simulink model "HEV_BTP_basic_Perfect_PID_17_1_2020"  (R2019a)
settings: Solver=VariableStepAuto  StartTime=0  StopTime=600  RelTol=1e-3
undefined symbols (not defined in the file): f_co, f_co2, f_hc, f_nox, f_tbrake_n_bpt, f_tbrake_t_bpt
libraries: nesl_utility x24, sdl_lib x16, fl_lib x13, simulink x6, autolibshared x1
settings Model: Creator=hp  LastModifiedBy=hp
settings SolverCC: ZeroCrossAlgorithm=Adaptive
settings DataIOCC: ExternalInput=[PedalTime,ThrottlePedal,FrontBrakePedal,RearBrakePedal]  LoadExternalInput=on
settings DebuggingCC: IgnoredZcDiagnostic=none

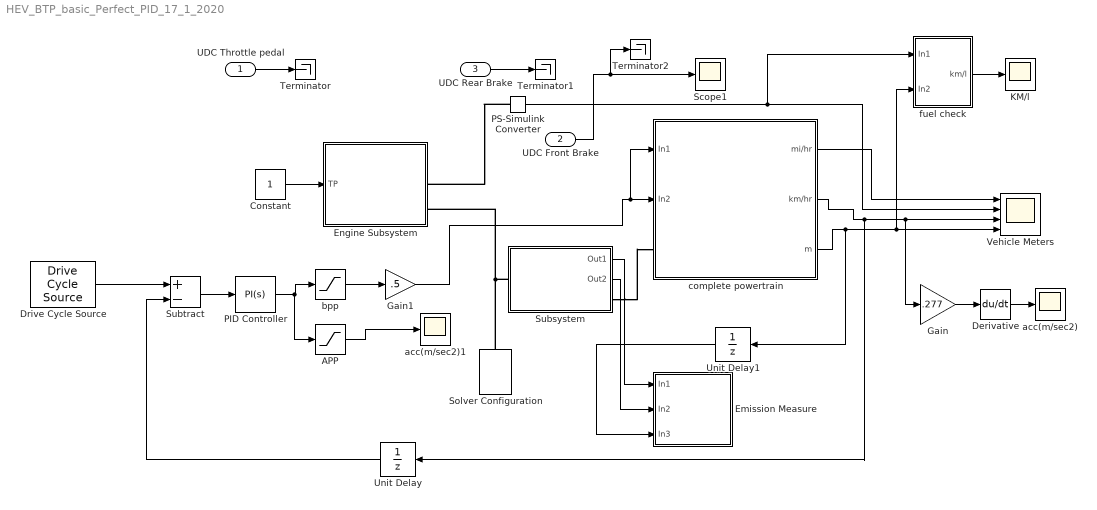
== system HEV_BTP_basic_Perfect_PID_17_1_2020 ==
  UDC Throttle pedal : Inport
  UDC Front Brake : Inport  Port=2
  UDC Rear Brake : Inport  Port=3
  APP : Saturate  UpperLimit=inf  LowerLimit=0
  Constant : Constant
  Derivative : Derivative
  Drive Cycle Source : autolibshared/Drive Cycle Source  cycleVar=US06  fileVar=cycleFTP75.mat  tfinal="600  seconds, Cyclic"  cycleRepeat=on  outAccPort=off  outGearPort=off  gearList=No gear data  t_wot1=5  xdot_woto=0  xdot_wot1=30  t_wot2=20  xdot_wot2=0  t_wotend=30  srcUnit=m/s  outUnit=km/hr  srcAccUnit=m/s/s  outAccUnit=m/s^2  dt=0  aMode=2
      settings: SourceProductName=Powertrain Blockset  SourceProductBaseCode=PW
  Emission Measure : Subsystem
  Engine Subsystem : Subsystem
  Gain : Gain  Gain=.277
  Gain1 : Gain  Gain=.5
  KM/l : Scope
  PID Controller : simulink/Continuous/PID Controller  Controller=PI  Form=Parallel  TimeDomain=Continuous-time  SampleTime=-1  IntegratorMethod=Forward Euler  FilterMethod=Forward Euler  ControllerParametersSource=internal  P=.145  I=.015  D=0  UseFilter=on  N=100  TunerSelectOption=Transfer Function Based (PID Tuner App)  InitialConditionSource=internal  InitialConditionForIntegrator=0  InitialConditionForFilter=0  DifferentiatorICPrevScaledInput=0  ExternalReset=none  TrackingMode=off  Kt=1  LimitOutput=off  UpperSaturationLimit=inf  LowerSaturationLimit=-inf  LinearizeAsGain=on  AntiWindupMode=none  Kb=1  POutMin=[]  POutMax=[]  IOutMin=[]  IOutMax=[]  DOutMin=[]  DOutMax=[]  NOutMin=[]  NOutMax=[]  SumOutMin=[]  SumOutMax=[]  SaturationOutMin=[]  SaturationOutMax=[]  PParamMin=[]  PParamMax=[]  IParamMin=[]  IParamMax=[]  DParamMin=[]  DParamMax=[]  NParamMin=[]  NParamMax=[]  KbParamMin=[]  KbParamMax=[]  KtParamMin=[]  KtParamMax=[]  KbOutMin=[]  KbOutMax=[]  KtOutMin=[]  KtOutMax=[]  IntegratorOutMin=[]  IntegratorOutMax=[]  FilterOutMin=[]  FilterOutMax=[]  SumI1OutMin=[]  SumI1OutMax=[]  SumI2OutMin=[]  SumI2OutMax=[]  SumI3OutMin=[]  SumI3OutMax=[]  SumI4OutMin=[]  SumI4OutMax=[]  SumDOutMin=[]  SumDOutMax=[]  DifferentiatorOutMin=[]  DifferentiatorOutMax=[]  FilterDiffOutCoefMin=[]  FilterDiffOutCoefMax=[]  ReciprocalOutMin=[]  ReciprocalOutMax=[]  SumDenOutMin=[]  SumDenOutMax=[]  SumNumOutMin=[]  SumNumOutMax=[]  DivideOutMin=[]  DivideOutMax=[]  IntegratorContinuousStateAttributes=''  IntegratorStateMustResolveToSignalObject=off  IntegratorRTWStateStorageClass=Auto  FilterContinuousStateAttributes=''  FilterStateMustResolveToSignalObject=off  FilterRTWStateStorageClass=Auto  ParallelPVariant=InternalParameters  IdealPVariant=Disabled  IVariant=InternalParameters  DVariant=Disabled  IntegratorVariant=Continuous  SatVariant=Disabled  AWVariant=Passthrough  PCopyVariant=Disabled  TRVariant=Disabled  FdbkBlocksVariant=Forward  IdealPFdbkVariant=Disabled  SatFdbkVariant=Disabled  DerivativeFilterVariant=Disabled  NVariant=Disabled  NCopyVariant=Disabled_SignalSpec  FilterICVariant=Disabled  IntegratorICVariant=InternalICs  ExternalResetVariant=Disabled  TRSumVariant=Passthrough  SumFdbkVariant=Disabled  SumVariant=Sum_PI
  PS-Simulink Converter : nesl_utility/PS-Simulink Converter  PhysicalDomain=network_engine_domain  SubClassName=ps_output  LeftPortType=input  RightPortType=output  PseudoPeriodic=off  Frequencies=[]  Unit=g/s  AffineConversion=off
  Scope1 : Scope
  Solver Configuration : nesl_utility/Solver Configuration  PhysicalDomain=network_engine_domain  SubClassName=solver  LeftPortType=input  RightPortType=generic  Tones=[]  Harmonics=[]  SimulateNoise=off  Profile=off  UseLocalSampling=off  EnableSwitchedLinearOptims=on  FrequencyDomain=off  UseCCode=off  RelTol=0.001  AbsTol=1e-06  MinStep=1e-09  ToWorkspace=off  RevertToSquareIcSolve=off  NumHomotopyIterations=100  PhasorMode=off  PhasorModeNumHarmonics=1  DoDC=off  ResidualTolerance=1e-09  UseLocalSolver=off  LocalSolverChoice=NE_BACKWARD_EULER_ADVANCER  LocalSolverSampleTime=0.001  DoFixedCost=off  MaxNonlinIter=3  MaxModeIter=2  LinearAlgebra=auto  EquationFormulation=NE_TIME_EF  DelaysMemoryBudget=1024  AutomaticFiltering=on  FilteringTimeConstant=0.001  PartitionStorageMethod=AS_NEEDED  PartitionMemoryBudget=1024  PartitionMethod=ROBUST
  Subsystem : Subsystem
  Subtract : Sum  Inputs=+-
  Terminator : Terminator
  Terminator1 : Terminator
  Terminator2 : Terminator
  Unit Delay : UnitDelay  SampleTime=-1  HasFrameUpgradeWarning=on
  Unit Delay1 : UnitDelay  SampleTime=-1  HasFrameUpgradeWarning=on
  "Vehicle Meters " : Scope  NumInputPorts=4
  acc(m/sec2) : Scope
  acc(m/sec2)1 : Scope
  bpp : Saturate  UpperLimit=0  LowerLimit=-inf
  complete powertrain : Subsystem
  "fuel check " : Subsystem
  wires:
  complete powertrain/2(km/hr) -> Unit Delay/1, "Vehicle Meters "/3, Gain/1
  complete powertrain/1(mi/hr) -> "Vehicle Meters "/1
  complete powertrain/3(m) -> Unit Delay1/1, "Vehicle Meters "/4, "fuel check "/2(In2)
  UDC Front Brake/1 -> Terminator2/1, Scope1/1
  PS-Simulink Converter/1 -> "fuel check "/1(In1), "Vehicle Meters "/2
  Subsystem/2(Out2) -> Emission Measure/2(In2)
  Subsystem/1(Out1) -> Emission Measure/1(In1)
  Unit Delay1/1 -> Emission Measure/3(In3)
  "fuel check "/1(km/l) -> KM/l/1
  Gain/1 -> Derivative/1
  Derivative/1 -> acc(m/sec2)/1
  Drive Cycle Source/1 -> Subtract/1
  Subtract/1 -> PID Controller/1
  PID Controller/1 -> APP/1, bpp/1
  bpp/1 -> Gain1/1
  Gain1/1 -> complete powertrain/1(In1), complete powertrain/2(In2)
  UDC Throttle pedal/1 -> Terminator/1
  UDC Rear Brake/1 -> Terminator1/1
  Unit Delay/1 -> Subtract/2
  APP/1 -> acc(m/sec2)1/1
  Constant/1 -> Engine Subsystem/1(TP)
  connections:
  Solver Configuration/RConn1 -- Engine Subsystem/RConn3 -- Subsystem/LConn1
  PS-Simulink Converter/LConn1 -- Engine Subsystem/RConn2
  Subsystem/RConn1 -- complete powertrain/LConn1

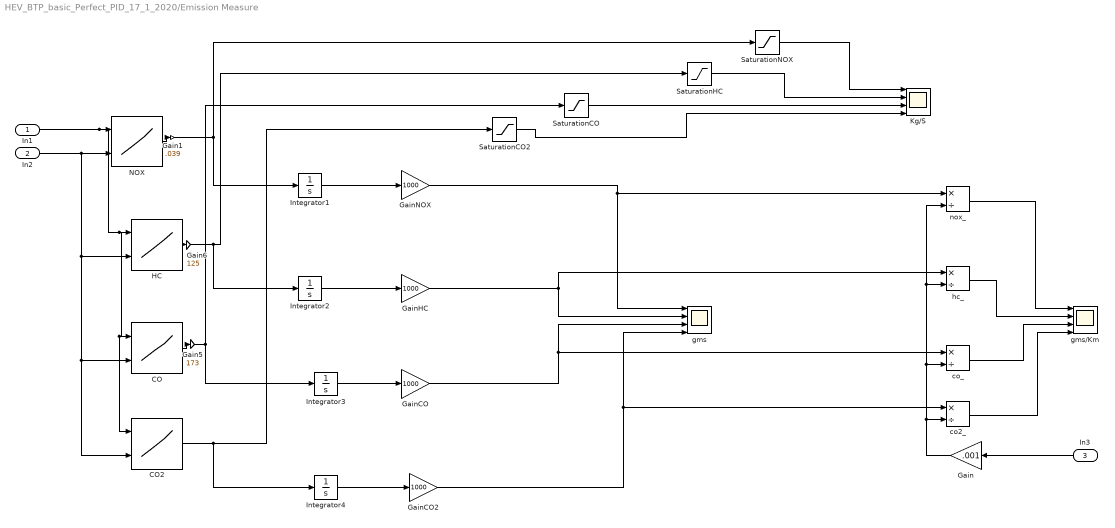
== system HEV_BTP_basic_Perfect_PID_17_1_2020/Emission Measure ==
  In1 : Inport
  In2 : Inport  Port=2
  In3 : Inport  Port=3
  CO : Lookup_n-D  BreakpointsForDimension1=f_tbrake_t_bpt  BreakpointsForDimension2=f_tbrake_n_bpt  Table=f_co  InternalRulePriority=Speed  RndMeth=Simplest  InputSameDT=on
  CO2 : Lookup_n-D  BreakpointsForDimension1=f_tbrake_t_bpt  BreakpointsForDimension2=f_tbrake_n_bpt  Table=f_co2  InternalRulePriority=Speed  RndMeth=Simplest  InputSameDT=on
  Gain : Gain  Gain=.001
  Gain1 : Gain  Gain=.039
  Gain5 : Gain  Gain=173
  Gain6 : Gain  Gain=125
  GainCO : Gain  Gain=1000
  GainCO2 : Gain  Gain=1000
  GainHC : Gain  Gain=1000
  GainNOX : Gain  Gain=1000
  HC : Lookup_n-D  BreakpointsForDimension1=f_tbrake_t_bpt  BreakpointsForDimension2=f_tbrake_n_bpt  Table=f_hc  InternalRulePriority=Speed  RndMeth=Simplest  InputSameDT=on
  Integrator{1..4} (4 alike) : Integrator
  Kg/S : Scope  NumInputPorts=4
  NOX : Lookup_n-D  BreakpointsForDimension1=f_tbrake_t_bpt  BreakpointsForDimension2=f_tbrake_n_bpt  Table=f_nox  InternalRulePriority=Speed  RndMeth=Simplest  InputSameDT=on
  SaturationCO : Saturate  UpperLimit=inf  LowerLimit=0  ZeroCross=off
  SaturationCO2 : Saturate  UpperLimit=inf  LowerLimit=0  ZeroCross=off
  SaturationHC : Saturate  UpperLimit=inf  LowerLimit=0  ZeroCross=off
  SaturationNOX : Saturate  UpperLimit=inf  LowerLimit=0  ZeroCross=off
  co2_ : Product  Inputs=*/
  co_ : Product  Inputs=*/
  gms : Scope  NumInputPorts=4
  gms/Km : Scope  NumInputPorts=4
  hc_ : Product  Inputs=*/
  nox_ : Product  Inputs=*/
  wires:
  NOX/1 -> Gain1/1
  In2/1 -> CO2/2, CO/2, HC/2, NOX/2
  In1/1 -> CO2/1, CO/1, HC/1, NOX/1
  HC/1 -> Gain6/1
  CO/1 -> Gain5/1
  CO2/1 -> SaturationCO2/1, Integrator4/1
  SaturationNOX/1 -> Kg/S/1
  SaturationHC/1 -> Kg/S/2
  SaturationCO2/1 -> Kg/S/4
  SaturationCO/1 -> Kg/S/3
  Gain6/1 -> Integrator2/1, SaturationHC/1
  Gain5/1 -> Integrator3/1, SaturationCO/1
  Integrator3/1 -> GainCO/1
  Integrator4/1 -> GainCO2/1
  Integrator2/1 -> GainHC/1
  Integrator1/1 -> GainNOX/1
  GainCO2/1 -> co2_/1, gms/4
  GainHC/1 -> gms/2, hc_/1
  GainNOX/1 -> nox_/1, gms/1
  GainCO/1 -> gms/3, co_/1
  Gain/1 -> nox_/2, hc_/2, co_/2, co2_/2
  nox_/1 -> gms/Km/1
  hc_/1 -> gms/Km/2
  co_/1 -> gms/Km/3
  co2_/1 -> gms/Km/4
  Gain1/1 -> Integrator1/1, SaturationNOX/1
  In3/1 -> Gain/1

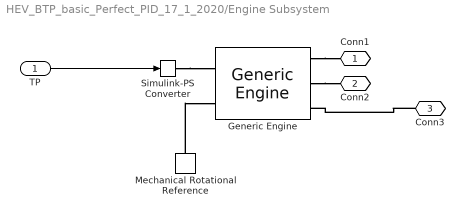
== system HEV_BTP_basic_Perfect_PID_17_1_2020/Engine Subsystem ==
  TP : Inport
  Generic Engine : sdl_lib/Engines/Generic Engine  model_parameterization=1  engine_type=1  P_max=51.5 kW  w_P_max=5500 rpm  w_max=6175 rpm  w_min=500 rpm  w_tab=[500, 1000, 2000, 3000, 4000, 5000, 6000, 7000] rpm  trq_tab=[380, 380, 380, 380, 350, 280, 200, 80] N*m  pwr_tab=[20, 40, 78, 120, 145, 148, 125, 60] kW  interp_method=simscape.enum.interpolation.linear  model_inertia=1  inertia=1 kg*m^2  initial_velocity=875 rpm  model_time_constant=1  time_constant=0.2 s  T0=.01  w_thr=100 rpm  idle_speed=0  idle_speed_reference=875 rpm  tau_controller=1 s  idle_w_thr=1 rpm  redline=0  redline_speed=5000 rpm  tau_redline=1 s  redline_w_thr=1 rpm  fc_model=2  fc_per_rev=22.816 mg/rev  displaced_volume=400 cm^3  rev_per_cycle=2  fc_w_tab=[875, 2000, 3000, 4000, 5000, 6175] rpm  fc_trq_tab=[0, 80, 160, 200, 240, 320, 360, 400] N*m  fc_tab=[0.2, 0.36, 0.56, 0.64, 0.76, 1.08, 1.36, 1.76; 0.4, 0.68, 1.08, 1.24, 1.44, 2, 2.4, 1.96; 0.56, 1.08, 1.6, 1.92, 2.24, 3, 3.4, 4.2; 0.8, 1.44, 2.32, 2.68, 3.2, 4.28, 4.68, 5.32; 1, 1.92, 3.16, 3.76, 4.32, 5.6, 6.48, 7.44; 1.24, 2.4, 4.12, 4.76, 5.52, 7.36, 8.8, 10.6] g/s  bmep_tab=[0, 250, 500, 625, 750, 1000, 1150, 1250] kPa  bsfc_tab=[410, 380, 300, 280, 270, 290, 320, 380; 410, 370, 290, 270, 260, 270, 285, 320; 415, 380, 290, 275, 265, 270, 270, 300; 420, 390, 310, 290, 285, 280, 280, 285; 430, 410, 340, 320, 310, 300, 310, 320; 450, 430, 370, 340, 330, 330, 350, 380] g/hr/kW  fc_interp_method=simscape.enum.interpolation.linear
      settings: SourceProductName=Simscape Driveline  SourceProductBaseCode=LD  LogSimulationData=on
  Mechanical Rotational Reference : fl_lib/Mechanical/Rotational Elements/Mechanical Rotational Reference
  Simulink-PS Converter : nesl_utility/Simulink-PS Converter  PhysicalDomain=network_engine_domain  SubClassName=ps_input  LeftPortType=input  RightPortType=output  PseudoPeriodic=off  Frequencies=[]  NoiseDistribution=none  NoiseParameters=[]  Unit=1  AffineConversion=off  FilteringAndDerivatives=provide  SimscapeFilterOrder=1  InputFilterTimeConstant=0.001  UdotUserProvided=0
  Conn1 : PMIOPort  Side=Right
  Conn2 : PMIOPort  Port=2  Side=Right
  Conn3 : PMIOPort  Port=3  Side=Right
  wires:
  TP/1 -> Simulink-PS Converter/1
  connections:
  Simulink-PS Converter/RConn1 -- Generic Engine/LConn1
  Generic Engine/RConn1 -- Conn1/RConn1
  Mechanical Rotational Reference/LConn1 -- Generic Engine/LConn2
  Conn3/RConn1 -- Generic Engine/RConn3
  Generic Engine/RConn2 -- Conn2/RConn1

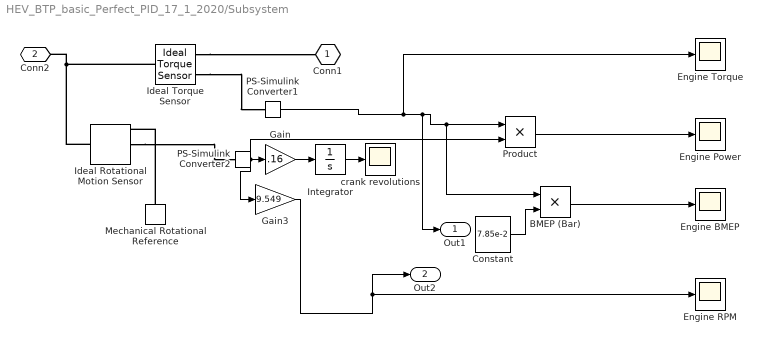
== system HEV_BTP_basic_Perfect_PID_17_1_2020/Subsystem ==
  BMEP (Bar) : Product
  Constant : Constant  Value=7.85e-2
  Engine BMEP : Scope
  Engine Power : Scope
  Engine Torque : Scope
  Engine RPM : Scope
  Gain : Gain  Gain=.16
  Gain3 : Gain  Gain=9.549
  Ideal Rotational Motion Sensor : fl_lib/Mechanical/Mechanical Sensors/Ideal Rotational Motion Sensor  offset=0 rad
  Ideal Torque Sensor : fl_lib/Mechanical/Mechanical Sensors/Ideal Torque Sensor
  Integrator : Integrator
  Mechanical Rotational Reference : fl_lib/Mechanical/Rotational Elements/Mechanical Rotational Reference
  PS-Simulink Converter1 : nesl_utility/PS-Simulink Converter  PhysicalDomain=network_engine_domain  SubClassName=ps_output  LeftPortType=input  RightPortType=output  PseudoPeriodic=off  Frequencies=[]  Unit=N*m  AffineConversion=off
  PS-Simulink Converter2 : nesl_utility/PS-Simulink Converter  PhysicalDomain=network_engine_domain  SubClassName=ps_output  LeftPortType=input  RightPortType=output  PseudoPeriodic=off  Frequencies=[]  Unit=rad/s  AffineConversion=off
  Product : Product
  crank revolutions : Scope
  Conn1 : PMIOPort  Side=Right
  Conn2 : PMIOPort  Port=2  Side=Left
  Out1 : Outport
  Out2 : Outport  Port=2
  wires:
  PS-Simulink Converter2/1 -> Product/2, Gain3/1, Gain/1
  Product/1 -> Engine Power/1
  PS-Simulink Converter1/1 -> Out1/1, BMEP (Bar)/1, Product/1, Engine Torque/1
  Gain/1 -> Integrator/1
  Integrator/1 -> crank revolutions/1
  Gain3/1 -> Out2/1, Engine RPM/1
  Constant/1 -> BMEP (Bar)/2
  BMEP (Bar)/1 -> Engine BMEP/1
  connections:
  Ideal Rotational Motion Sensor/LConn1 -- Conn2/RConn1 -- Ideal Torque Sensor/LConn1
  Mechanical Rotational Reference/LConn1 -- Ideal Rotational Motion Sensor/RConn1
  Ideal Torque Sensor/RConn2 -- PS-Simulink Converter1/LConn1
  Ideal Torque Sensor/RConn1 -- Conn1/RConn1
  Ideal Rotational Motion Sensor/RConn2 -- PS-Simulink Converter2/LConn1

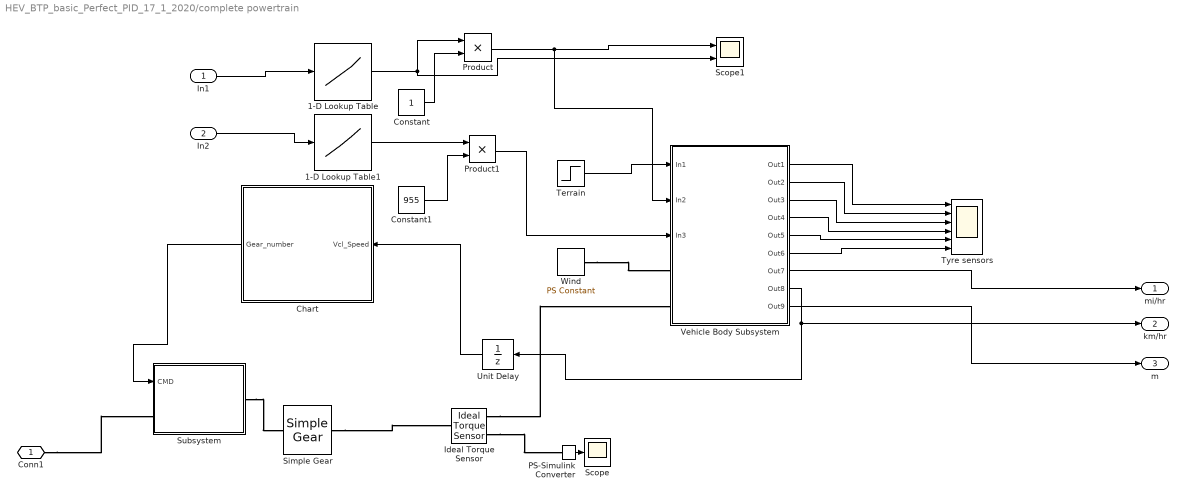
== system HEV_BTP_basic_Perfect_PID_17_1_2020/complete powertrain ==
  In1 : Inport
  In2 : Inport  Port=2
  1-D Lookup Table : Lookup_n-D  NumberOfTableDimensions=1  BreakpointsForDimension1=0:0.01:1  Table=0:10:1000  InternalRulePriority=Speed  RndMeth=Simplest  InputSameDT=on
  1-D Lookup Table1 : Lookup_n-D  NumberOfTableDimensions=1  BreakpointsForDimension1=0:0.01:1  Table=0:10:1000  InternalRulePriority=Speed  RndMeth=Simplest  InputSameDT=on
  Chart : Stateflow chart  BlockKeywords=__PRM__SERIALIZED__DATA__:Stateflow Chart,Stateflow Diagram  TreatAsAtomicUnit=on
  Constant : Constant
  Constant1 : Constant  Value=955
  Ideal Torque Sensor : fl_lib/Mechanical/Mechanical Sensors/Ideal Torque Sensor
  PS-Simulink Converter : nesl_utility/PS-Simulink Converter  PhysicalDomain=network_engine_domain  SubClassName=ps_output  LeftPortType=input  RightPortType=output  PseudoPeriodic=off  Frequencies=[]  Unit=N*m  AffineConversion=off
  Product : Product
  Product1 : Product
  Scope : Scope
  Scope1 : Scope  NumInputPorts=2
  Simple Gear : sdl_lib/Gears/Simple Gear  ratio=6  rotation_direction=1  friction_model=sdl.enum.gear_efficiencies_load.off  T_noload=0.1 N*m  T_nom=5 N*m  efficiency_nom=0.8  efficiency=0.8  mu_visc=[0, 0] N*m/(rad/s)  w_thr=0.01 rad/s  pwr_thr=0.001 W  enable_faults=simscape.enum.onoff.off  efficiency_fault=0.05  external_fault=simscape.enum.onoff.off  temporal_fault=simscape.enum.onoff.off  fault_time=5 s  fault_angles=pi / 12 rad  report_fault=1  temperature_TLU=[280, 300, 320] K  load_TLU=[1, 5, 10] N*m  efficiency_TLU=[.95, .9, .85]  efficiency_TLU2=[.85, .8, .75; .95, .9, .85; .85, .8, .7]  thermal_mass=50 J/K  T_init=300 K
      settings: SourceProductName=Simscape Driveline
  Subsystem : Subsystem
  Terrain : Step  Time=700  Before=-0.5*(pi/180)  After=0  SampleTime=0
  Tyre sensors : Scope  NumInputPorts=6
  Unit Delay : UnitDelay  SampleTime=.05  HasFrameUpgradeWarning=on
  Vehicle Body Subsystem : Subsystem
  "Wind " : fl_lib/Physical Signals/Sources/PS Constant  constant=3 m/s
  Conn1 : PMIOPort  Side=Left
  mi/hr : Outport
  km/hr : Outport  Port=2
  m : Outport  Port=3
  wires:
  Terrain/1 -> Vehicle Body Subsystem/1(In1)
  Vehicle Body Subsystem/1(Out1) -> Tyre sensors/1
  Vehicle Body Subsystem/3(Out3) -> Tyre sensors/3
  Vehicle Body Subsystem/6(Out6) -> Tyre sensors/6
  Vehicle Body Subsystem/5(Out5) -> Tyre sensors/5
  Vehicle Body Subsystem/2(Out2) -> Tyre sensors/2
  PS-Simulink Converter/1 -> Scope/1
  Vehicle Body Subsystem/4(Out4) -> Tyre sensors/4
  Chart/1(Gear_number) -> Subsystem/1("CMD ")
  Vehicle Body Subsystem/8(Out8) -> km/hr/1, Unit Delay/1
  Unit Delay/1 -> Chart/1(Vcl_Speed)
  Vehicle Body Subsystem/7(Out7) -> mi/hr/1
  Vehicle Body Subsystem/9(Out9) -> m/1
  In1/1 -> 1-D Lookup Table/1
  In2/1 -> 1-D Lookup Table1/1
  1-D Lookup Table/1 -> Product/1, Scope1/2
  Constant/1 -> Product/2
  Product/1 -> Vehicle Body Subsystem/2(In2), Scope1/1
  1-D Lookup Table1/1 -> Product1/1
  Constant1/1 -> Product1/2
  Product1/1 -> Vehicle Body Subsystem/3(In3)
  connections:
  Ideal Torque Sensor/RConn1 -- Vehicle Body Subsystem/LConn2
  "Wind "/RConn1 -- Vehicle Body Subsystem/LConn1
  Subsystem/RConn1 -- Simple Gear/LConn1
  Ideal Torque Sensor/RConn2 -- PS-Simulink Converter/LConn1
  Conn1/RConn1 -- Subsystem/LConn1
  Simple Gear/RConn1 -- Ideal Torque Sensor/LConn1

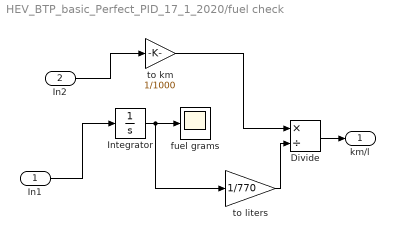
== system HEV_BTP_basic_Perfect_PID_17_1_2020/fuel check  ==
  In1 : Inport
  In2 : Inport  Port=2
  Divide : Product  Inputs=*/
  Integrator : Integrator
  fuel grams : Scope
  to km : Gain  Gain=1/1000
  to liters : Gain  Gain=1/770
  km/l : Outport
  wires:
  Integrator/1 -> to liters/1, fuel grams/1
  In2/1 -> to km/1
  to liters/1 -> Divide/2
  Divide/1 -> km/l/1
  In1/1 -> Integrator/1
  to km/1 -> Divide/1

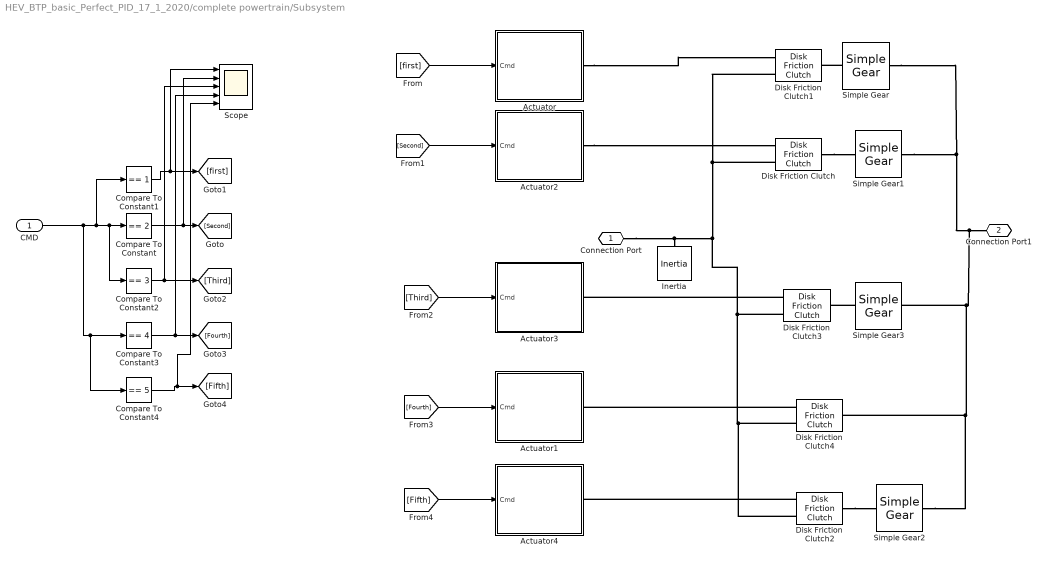
== system HEV_BTP_basic_Perfect_PID_17_1_2020/complete powertrain/Subsystem ==
  "CMD " : Inport
  Actuator : Subsystem
  Actuator1 : Subsystem
  Actuator2 : Subsystem
  Actuator3 : Subsystem
  Actuator4 : Subsystem
  Compare To Constant : simulink/Logic and Bit Operations/Compare To Constant  relop===  const=2  OutDataTypeStr=boolean
  Compare To Constant1 : simulink/Logic and Bit Operations/Compare To Constant  relop===  const=1  OutDataTypeStr=boolean
  Compare To Constant2 : simulink/Logic and Bit Operations/Compare To Constant  relop===  const=3  OutDataTypeStr=boolean
  Compare To Constant3 : simulink/Logic and Bit Operations/Compare To Constant  relop===  const=4  OutDataTypeStr=boolean
  Compare To Constant4 : simulink/Logic and Bit Operations/Compare To Constant  relop===  const=5  OutDataTypeStr=boolean
  Disk Friction Clutch{,1..4} (5 alike) : sdl_lib/Clutches/Disk Friction Clutch  geometry_model=1  r_eff=130 mm  d_o=150 mm  d_i=100 mm  nS=4  piston_area=0.001 m^2  unidirectional=0  friction_model=1  mu_coulomb=0.3  mu_w_vector=[0, 100, 1000] rad/s  mu_coulomb_vector=[.3, .22, .19]  mu_interp_method=simscape.enum.interpolation.linear  mu_extrap_method=simscape.enum.extrapolation.linear  mu_static=0.35  d_f=1  w_tol=0.001 rad/s  pressure_min=100 Pa  mu_visc=0 N*m/(rad/s)  initial_state_locked=0  temperature_TLU=[280, 300, 320] K  mu_coulomb_temp_vector=[.3, .28, .25]  mu_coulomb_matrix=[.34, .32, .3; .3, .28, .25; .25, .2, .15]  mu_static_vector=[.4, .38, .36]  thermal_mass=25 kJ/K  T_init=300 K
      settings: SourceProductName=Simscape Driveline  SourceProductBaseCode=LD
  Inertia : fl_lib/Mechanical/Rotational Elements/Inertia  inertia=0.01 kg*m^2  w_specify=on  w_priority=None  w=0 rad/s  w_nominal_specify=off  w_nominal_unit=rad/s  w_nominal_value=1  t_specify=off  t_priority=None  t=0 N*m  t_nominal_specify=off  t_nominal_unit=N*m  t_nominal_value=1
  Scope : Scope  NumInputPorts=5
  Simple Gear : sdl_lib/Gears/Simple Gear  ratio=2.95  rotation_direction=1  friction_model=sdl.enum.gear_efficiencies_load.off  T_noload=0.1 N*m  T_nom=5 N*m  efficiency_nom=0.8  efficiency=0.8  mu_visc=[0, 0] N*m/(rad/s)  w_thr=0.01 rad/s  pwr_thr=0.001 W  enable_faults=simscape.enum.onoff.off  efficiency_fault=0.05  external_fault=simscape.enum.onoff.off  temporal_fault=simscape.enum.onoff.off  fault_time=5 s  fault_angles=pi / 12 rad  report_fault=1  temperature_TLU=[280, 300, 320] K  load_TLU=[1, 5, 10] N*m  efficiency_TLU=[.95, .9, .85]  efficiency_TLU2=[.85, .8, .75; .95, .9, .85; .85, .8, .7]  thermal_mass=50 J/K  T_init=300 K
      settings: SourceProductName=Simscape Driveline
  Simple Gear1 : sdl_lib/Gears/Simple Gear  ratio=1.94  rotation_direction=1  friction_model=sdl.enum.gear_efficiencies_load.off  T_noload=0.1 N*m  T_nom=5 N*m  efficiency_nom=0.8  efficiency=0.8  mu_visc=[0, 0] N*m/(rad/s)  w_thr=0.01 rad/s  pwr_thr=0.001 W  enable_faults=simscape.enum.onoff.off  efficiency_fault=0.05  external_fault=simscape.enum.onoff.off  temporal_fault=simscape.enum.onoff.off  fault_time=5 s  fault_angles=pi / 12 rad  report_fault=1  temperature_TLU=[280, 300, 320] K  load_TLU=[1, 5, 10] N*m  efficiency_TLU=[.95, .9, .85]  efficiency_TLU2=[.85, .8, .75; .95, .9, .85; .85, .8, .7]  thermal_mass=50 J/K  T_init=300 K
      settings: SourceProductName=Simscape Driveline
  Simple Gear2 : sdl_lib/Gears/Simple Gear  ratio=.68  rotation_direction=1  friction_model=sdl.enum.gear_efficiencies_load.off  T_noload=0.1 N*m  T_nom=5 N*m  efficiency_nom=0.8  efficiency=0.8  mu_visc=[0, 0] N*m/(rad/s)  w_thr=0.01 rad/s  pwr_thr=0.001 W  enable_faults=simscape.enum.onoff.off  efficiency_fault=0.05  external_fault=simscape.enum.onoff.off  temporal_fault=simscape.enum.onoff.off  fault_time=5 s  fault_angles=pi / 12 rad  report_fault=1  temperature_TLU=[280, 300, 320] K  load_TLU=[1, 5, 10] N*m  efficiency_TLU=[.95, .9, .85]  efficiency_TLU2=[.85, .8, .75; .95, .9, .85; .85, .8, .7]  thermal_mass=50 J/K  T_init=300 K
      settings: SourceProductName=Simscape Driveline
  Simple Gear3 : sdl_lib/Gears/Simple Gear  ratio=1.34  rotation_direction=1  friction_model=sdl.enum.gear_efficiencies_load.off  T_noload=0.1 N*m  T_nom=5 N*m  efficiency_nom=0.8  efficiency=0.8  mu_visc=[0, 0] N*m/(rad/s)  w_thr=0.01 rad/s  pwr_thr=0.001 W  enable_faults=simscape.enum.onoff.off  efficiency_fault=0.05  external_fault=simscape.enum.onoff.off  temporal_fault=simscape.enum.onoff.off  fault_time=5 s  fault_angles=pi / 12 rad  report_fault=1  temperature_TLU=[280, 300, 320] K  load_TLU=[1, 5, 10] N*m  efficiency_TLU=[.95, .9, .85]  efficiency_TLU2=[.85, .8, .75; .95, .9, .85; .85, .8, .7]  thermal_mass=50 J/K  T_init=300 K
      settings: SourceProductName=Simscape Driveline
  Connection Port : PMIOPort  Side=Left
  Connection Port1 : PMIOPort  Port=2  Side=Right
  wires:
  Compare To Constant/1 -> Scope/2, [Second]
  [first] -> Actuator/1(Cmd)
  Compare To Constant1/1 -> Scope/1, [first]
  Compare To Constant2/1 -> Scope/3, [Third]
  Compare To Constant3/1 -> Scope/4, [Fourth]
  "CMD "/1 -> Compare To Constant2/1, Compare To Constant/1, Compare To Constant1/1, Compare To Constant4/1, Compare To Constant3/1
  [Second] -> Actuator2/1(Cmd)
  [Third] -> Actuator3/1(Cmd)
  [Fourth] -> Actuator1/1(Cmd)
  Compare To Constant4/1 -> Scope/5, [Fifth]
  [Fifth] -> Actuator4/1(Cmd)
  connections:
  Disk Friction Clutch/RConn1 -- Simple Gear1/LConn1
  Disk Friction Clutch/LConn2 -- Inertia/LConn1 -- Connection Port/RConn1 -- Disk Friction Clutch2/LConn2 -- Disk Friction Clutch4/LConn2 -- Disk Friction Clutch3/LConn2 -- Disk Friction Clutch1/LConn2
  Actuator/RConn1 -- Disk Friction Clutch1/LConn1
  Actuator2/RConn1 -- Disk Friction Clutch/LConn1
  Disk Friction Clutch3/LConn1 -- Actuator3/RConn1
  Disk Friction Clutch4/LConn1 -- Actuator1/RConn1
  Simple Gear/LConn1 -- Disk Friction Clutch1/RConn1
  Simple Gear1/RConn1 -- Simple Gear/RConn1 -- Disk Friction Clutch4/RConn1 -- Simple Gear2/RConn1 -- Simple Gear3/RConn1 -- Connection Port1/RConn1
  Disk Friction Clutch2/RConn1 -- Simple Gear2/LConn1
  Disk Friction Clutch2/LConn1 -- Actuator4/RConn1
  Simple Gear3/LConn1 -- Disk Friction Clutch3/RConn1

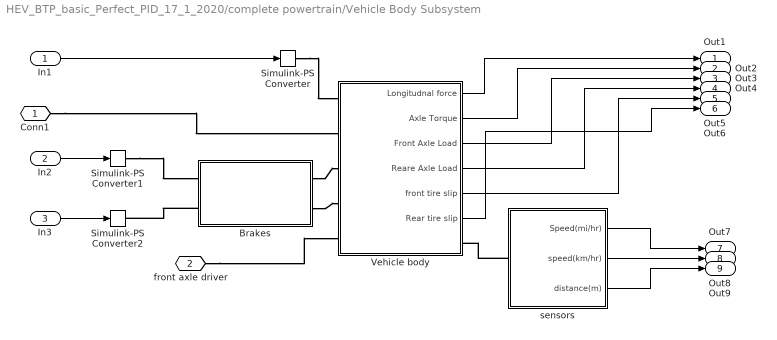
== system HEV_BTP_basic_Perfect_PID_17_1_2020/complete powertrain/Vehicle Body Subsystem ==
  In1 : Inport
  In2 : Inport  Port=2
  In3 : Inport  Port=3
  Brakes : Subsystem
  Simulink-PS Converter : nesl_utility/Simulink-PS Converter  PhysicalDomain=network_engine_domain  SubClassName=ps_input  LeftPortType=input  RightPortType=output  PseudoPeriodic=off  Frequencies=[]  NoiseDistribution=none  NoiseParameters=[]  Unit=1  AffineConversion=off  FilteringAndDerivatives=provide  SimscapeFilterOrder=1  InputFilterTimeConstant=0.001  UdotUserProvided=0
  Simulink-PS Converter1 : nesl_utility/Simulink-PS Converter  PhysicalDomain=network_engine_domain  SubClassName=ps_input  LeftPortType=input  RightPortType=output  PseudoPeriodic=off  Frequencies=[]  NoiseDistribution=none  NoiseParameters=[]  Unit=N  AffineConversion=off  FilteringAndDerivatives=provide  SimscapeFilterOrder=1  InputFilterTimeConstant=0.001  UdotUserProvided=0
  Simulink-PS Converter2 : nesl_utility/Simulink-PS Converter  PhysicalDomain=network_engine_domain  SubClassName=ps_input  LeftPortType=input  RightPortType=output  PseudoPeriodic=off  Frequencies=[]  NoiseDistribution=none  NoiseParameters=[]  Unit=N  AffineConversion=off  FilteringAndDerivatives=provide  SimscapeFilterOrder=1  InputFilterTimeConstant=0.001  UdotUserProvided=0
  Vehicle body : Subsystem
  sensors : Subsystem
  Conn1 : PMIOPort  Side=Left
  front axle driver : PMIOPort  Port=2  Side=Left
  Out1 : Outport
  Out2 : Outport  Port=2
  Out3 : Outport  Port=3
  Out4 : Outport  Port=4
  Out5 : Outport  Port=5
  Out6 : Outport  Port=6
  Out7 : Outport  Port=7
  Out8 : Outport  Port=8
  Out9 : Outport  Port=9
  wires:
  Vehicle body/1(Longitudnal force) -> Out1/1
  Vehicle body/2(Axle Torque) -> Out2/1
  sensors/1(Speed(mi/hr)) -> Out7/1
  Vehicle body/5(front tire slip) -> Out5/1
  Vehicle body/6(Rear tire slip) -> Out6/1
  sensors/2(speed(km/hr)) -> Out8/1
  In1/1 -> Simulink-PS Converter/1
  In3/1 -> Simulink-PS Converter2/1
  sensors/3("distance(m) ") -> Out9/1
  In2/1 -> Simulink-PS Converter1/1
  Vehicle body/3(Front Axle Load) -> Out3/1
  Vehicle body/4(Reare Axle Load) -> Out4/1
  connections:
  Simulink-PS Converter1/RConn1 -- Brakes/LConn1
  Brakes/LConn2 -- Simulink-PS Converter2/RConn1
  sensors/LConn1 -- Vehicle body/RConn1
  Brakes/RConn1 -- Vehicle body/LConn3
  Brakes/RConn2 -- Vehicle body/LConn4
  Simulink-PS Converter/RConn1 -- Vehicle body/LConn1
  Conn1/RConn1 -- Vehicle body/LConn2
  front axle driver/RConn1 -- Vehicle body/LConn5

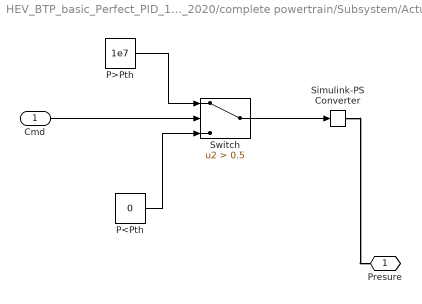
== system HEV_BTP_basic_Perfect_PID_17_1_2020/complete powertrain/Subsystem/Actuator ==
  Cmd : Inport
  P<Pth : Constant  Value=0
  P>Pth : Constant  Value=1e7
  Simulink-PS Converter : nesl_utility/Simulink-PS Converter  PhysicalDomain=network_engine_domain  SubClassName=ps_input  LeftPortType=input  RightPortType=output  PseudoPeriodic=off  Frequencies=[]  NoiseDistribution=none  NoiseParameters=[]  Unit=1  AffineConversion=off  FilteringAndDerivatives=provide  SimscapeFilterOrder=1  InputFilterTimeConstant=0.001  UdotUserProvided=0
  Switch : Switch  Criteria=u2 > Threshold  Threshold=0.5
  Presure : PMIOPort  Side=Right
  wires:
  Cmd/1 -> Switch/2
  Switch/1 -> Simulink-PS Converter/1
  P<Pth/1 -> Switch/3
  P>Pth/1 -> Switch/1
  connections:
  Simulink-PS Converter/RConn1 -- Presure/RConn1

== system HEV_BTP_basic_Perfect_PID_17_1_2020/complete powertrain/Subsystem/Actuator1 ==
  Cmd : Inport
  P<Pth : Constant  Value=0
  P>Pth : Constant  Value=1e7
  Simulink-PS Converter : nesl_utility/Simulink-PS Converter  PhysicalDomain=network_engine_domain  SubClassName=ps_input  LeftPortType=input  RightPortType=output  PseudoPeriodic=off  Frequencies=[]  NoiseDistribution=none  NoiseParameters=[]  Unit=1  AffineConversion=off  FilteringAndDerivatives=provide  SimscapeFilterOrder=1  InputFilterTimeConstant=0.001  UdotUserProvided=0
  Switch : Switch  Criteria=u2 > Threshold  Threshold=0.5
  Presure : PMIOPort  Side=Right
  wires:
  P>Pth/1 -> Switch/1
  P<Pth/1 -> Switch/3
  Switch/1 -> Simulink-PS Converter/1
  Cmd/1 -> Switch/2
  connections:
  Simulink-PS Converter/RConn1 -- Presure/RConn1

== system HEV_BTP_basic_Perfect_PID_17_1_2020/complete powertrain/Subsystem/Actuator2 ==
  Cmd : Inport
  P<Pth : Constant  Value=0
  P>Pth : Constant  Value=1e7
  Simulink-PS Converter : nesl_utility/Simulink-PS Converter  PhysicalDomain=network_engine_domain  SubClassName=ps_input  LeftPortType=input  RightPortType=output  PseudoPeriodic=off  Frequencies=[]  NoiseDistribution=none  NoiseParameters=[]  Unit=1  AffineConversion=off  FilteringAndDerivatives=provide  SimscapeFilterOrder=1  InputFilterTimeConstant=0.001  UdotUserProvided=0
  Switch : Switch  Criteria=u2 > Threshold  Threshold=.5
  Presure : PMIOPort  Side=Right
  wires:
  P>Pth/1 -> Switch/1
  P<Pth/1 -> Switch/3
  Switch/1 -> Simulink-PS Converter/1
  Cmd/1 -> Switch/2
  connections:
  Simulink-PS Converter/RConn1 -- Presure/RConn1

== system HEV_BTP_basic_Perfect_PID_17_1_2020/complete powertrain/Subsystem/Actuator3 ==
  Cmd : Inport
  P<Pth : Constant  Value=0
  P>Pth : Constant  Value=1e7
  Simulink-PS Converter : nesl_utility/Simulink-PS Converter  PhysicalDomain=network_engine_domain  SubClassName=ps_input  LeftPortType=input  RightPortType=output  PseudoPeriodic=off  Frequencies=[]  NoiseDistribution=none  NoiseParameters=[]  Unit=1  AffineConversion=off  FilteringAndDerivatives=provide  SimscapeFilterOrder=1  InputFilterTimeConstant=0.001  UdotUserProvided=0
  Switch : Switch  Criteria=u2 > Threshold  Threshold=0.5
  Presure : PMIOPort  Side=Right
  wires:
  P>Pth/1 -> Switch/1
  P<Pth/1 -> Switch/3
  Switch/1 -> Simulink-PS Converter/1
  Cmd/1 -> Switch/2
  connections:
  Simulink-PS Converter/RConn1 -- Presure/RConn1

== system HEV_BTP_basic_Perfect_PID_17_1_2020/complete powertrain/Subsystem/Actuator4 ==
  Cmd : Inport
  P<Pth : Constant  Value=0
  P>Pth : Constant  Value=1e7
  Simulink-PS Converter : nesl_utility/Simulink-PS Converter  PhysicalDomain=network_engine_domain  SubClassName=ps_input  LeftPortType=input  RightPortType=output  PseudoPeriodic=off  Frequencies=[]  NoiseDistribution=none  NoiseParameters=[]  Unit=1  AffineConversion=off  FilteringAndDerivatives=provide  SimscapeFilterOrder=1  InputFilterTimeConstant=0.001  UdotUserProvided=0
  Switch : Switch  Criteria=u2 > Threshold  Threshold=0.5
  Presure : PMIOPort  Side=Right
  wires:
  Cmd/1 -> Switch/2
  Switch/1 -> Simulink-PS Converter/1
  P<Pth/1 -> Switch/3
  P>Pth/1 -> Switch/1
  connections:
  Simulink-PS Converter/RConn1 -- Presure/RConn1

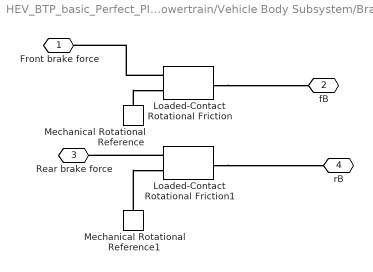
== system HEV_BTP_basic_Perfect_PID_17_1_2020/complete powertrain/Vehicle Body Subsystem/Brakes ==
  Loaded-Contact Rotational Friction : sdl_lib/Brakes & Detents/Rotational/Loaded-Contact Rotational Friction  geometry_model=1  r_eff=130 mm  d_o=150 mm  d_i=100 mm  friction_model=1  mu_coulomb=0.3  mu_w_vector=[0, 100, 1000] rad/s  mu_coulomb_vector=[.3, .22, .19]  mu_interp_method=simscape.enum.interpolation.linear  mu_extrap_method=simscape.enum.extrapolation.linear  mu_static=0.35  w_tol=0.001 rad/s  force_min=10 N  mu_visc=0 N*m/(rad/s)  initial_state_locked=0  temperature_TLU=[280, 300, 320] K  mu_coulomb_temp_vector=[.3, .28, .25]  mu_coulomb_matrix=[.34, .32, .3; .3, .28, .25; .25, .2, .15]  mu_static_vector=[.4, .38, .36]  thermal_mass=50 kJ/K  T_init=300 K
      settings: SourceProductName=Simscape Driveline  SourceProductBaseCode=LD
  Loaded-Contact Rotational Friction1 : sdl_lib/Brakes & Detents/Rotational/Loaded-Contact Rotational Friction  geometry_model=1  r_eff=130 mm  d_o=150 mm  d_i=100 mm  friction_model=1  mu_coulomb=0.3  mu_w_vector=[0, 100, 1000] rad/s  mu_coulomb_vector=[.3, .22, .19]  mu_interp_method=simscape.enum.interpolation.linear  mu_extrap_method=simscape.enum.extrapolation.linear  mu_static=0.35  w_tol=0.001 rad/s  force_min=10 N  mu_visc=0 N*m/(rad/s)  initial_state_locked=0  temperature_TLU=[280, 300, 320] K  mu_coulomb_temp_vector=[.3, .28, .25]  mu_coulomb_matrix=[.34, .32, .3; .3, .28, .25; .25, .2, .15]  mu_static_vector=[.4, .38, .36]  thermal_mass=50 kJ/K  T_init=300 K
      settings: SourceProductName=Simscape Driveline  SourceProductBaseCode=LD
  Mechanical Rotational Reference : fl_lib/Mechanical/Rotational Elements/Mechanical Rotational Reference
  Mechanical Rotational Reference1 : fl_lib/Mechanical/Rotational Elements/Mechanical Rotational Reference
  Front brake force : PMIOPort  Side=Left
  fB : PMIOPort  Port=2  Side=Right
  Rear brake force : PMIOPort  Port=3  Side=Left
  rB : PMIOPort  Port=4  Side=Right
  connections:
  Mechanical Rotational Reference1/LConn1 -- Loaded-Contact Rotational Friction1/LConn2
  Loaded-Contact Rotational Friction/RConn1 -- fB/RConn1
  Mechanical Rotational Reference/LConn1 -- Loaded-Contact Rotational Friction/LConn2
  Loaded-Contact Rotational Friction/LConn1 -- Front brake force/RConn1
  Loaded-Contact Rotational Friction1/RConn1 -- rB/RConn1
  Loaded-Contact Rotational Friction1/LConn1 -- Rear brake force/RConn1

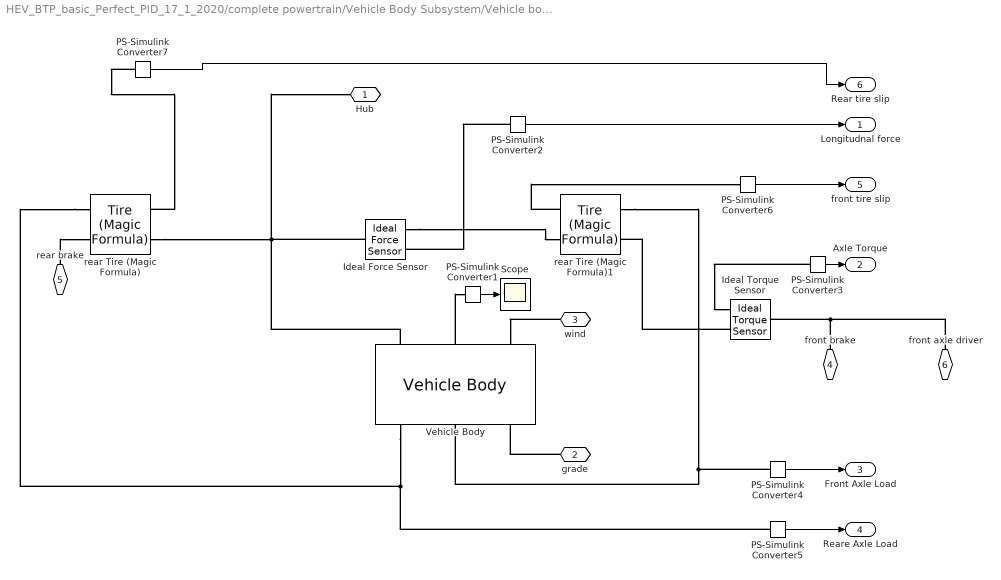
== system HEV_BTP_basic_Perfect_PID_17_1_2020/complete powertrain/Vehicle Body Subsystem/Vehicle body ==
  Ideal Force Sensor : fl_lib/Mechanical/Mechanical Sensors/Ideal Force Sensor
  Ideal Torque Sensor : fl_lib/Mechanical/Mechanical Sensors/Ideal Torque Sensor
  PS-Simulink Converter{1..7} (7 alike) : nesl_utility/PS-Simulink Converter  PhysicalDomain=network_engine_domain  SubClassName=ps_output  LeftPortType=input  RightPortType=output  PseudoPeriodic=off  Frequencies=[]  Unit=1  AffineConversion=off
  Scope : Scope
  Vehicle Body : sdl_lib/Tires & Vehicles/Vehicle Body  mass=1200 kg  n_w=1  x_f=1.160 m  x_r=1.325 m  y_c=0.5 m  mass_var=simscape.enum.onoff.off  model_pitch=simscape.enum.onoff.off  inertia=4000 kg*m^2  suspension_model=sdl.enum.linearTLU.linear  k_f=1e4 N/m  b_f=1e4 N/(m/s)  k_r=1e4 N/m  b_r=1e4 N/(m/s)  k_f_TLU=[-2000, -1000, 0, 1000, 2000] N  x_f_TLU=[-.4, -.2, 0, .2, .4] m  b_f_TLU=[-200, -100, 0, 100, 200] N  v_f_TLU=[-4, -2, 0, 2, 4] m/s  k_r_TLU=[-2000, -1000, 0, 1000, 2000] N  x_r_TLU=[-.4, -.2, 0, .2, .4] m  b_r_TLU=[-200, -100, 0, 100, 200] N  v_r_TLU=[-4, -2, 0, 2, 4] m/s  interp_method=simscape.enum.interpolation.linear  extrap_method=simscape.enum.extrapolation.linear  model_hardstop=simscape.enum.onoff.off  upper_bound_f=.25 m  lower_bound_f=-.25 m  stop_k_f=1e6 N/m  stop_b_f=150 N/(m/s)  upper_bound_r=.25 m  lower_bound_r=-.25 m  stop_k_r=1e6 N/m  stop_b_r=150 N/(m/s)  initial_pitch=0 rad  initial_pitch_rate=0 rad/s  g=9.81 m/s^2  liftoff_warning=simscape.enum.onoff.off  area=1.78 m^2  Cd=0.3  rho=1.225 kg/m^3  v_specify=off  v_priority=High  v=0 m/s  v_nominal_specify=off  v_nominal_unit=m/s  v_nominal_value=1
      settings: SourceProductName=Simscape Driveline
  rear Tire (Magic Formula) : sdl_lib/Tires & Vehicles/Tire (Magic Formula)  parameterization=sdl.enum.magic_tire_model.constant  F_z1=3000 N  F_x1=3500 N  kappa1=10  B_m=10  C_m=1.9  D_m=1  E_m=0.97  fz0=4000 N  p_Cx=1.685  p_Dx=[1.21, -.037]  p_Ex=[.344, .095, -.02, 0]  p_Kx=[21.51, -.163, .245]  p_Hx=[-.002, .002]  p_Vx=[0, 0]  v_tr_thr=0.1 m/s  r_e=.27 m  model_compliance=0  stiffness=1e6 N/m  damping=1000 N/(m/s)  model_inertia=1  inertia=.51 kg*m^2  initial_velocity=0 rad/s  model_resistance=1  resistance_model=1  coeff=0.015  p_tire=250e3 Pa  alpha=-0.003  beta=0.97  coeff_a=84e-4  coeff_b=6.2e-4 s/m  coeff_c=1.6e-4 s^2/m^2  v_thr=0.001 m/s
      settings: SourceProductName=Simscape Driveline
  rear Tire (Magic Formula)1 : sdl_lib/Tires & Vehicles/Tire (Magic Formula)  parameterization=sdl.enum.magic_tire_model.constant  F_z1=3000 N  F_x1=3500 N  kappa1=10  B_m=10  C_m=1.9  D_m=1  E_m=0.97  fz0=4000 N  p_Cx=1.685  p_Dx=[1.21, -.037]  p_Ex=[.344, .095, -.02, 0]  p_Kx=[21.51, -.163, .245]  p_Hx=[-.002, .002]  p_Vx=[0, 0]  v_tr_thr=0.1 m/s  r_e=.27 m  model_compliance=0  stiffness=1e6 N/m  damping=1000 N/(m/s)  model_inertia=1  inertia=.51 kg*m^2  initial_velocity=0 rad/s  model_resistance=1  resistance_model=1  coeff=0.015  p_tire=250e3 Pa  alpha=-0.003  beta=0.97  coeff_a=84e-4  coeff_b=6.2e-4 s/m  coeff_c=1.6e-4 s^2/m^2  v_thr=0.001 m/s
      settings: SourceProductName=Simscape Driveline
  Hub : PMIOPort  Side=Right
  grade : PMIOPort  Port=2  Side=Left
  wind : PMIOPort  Port=3  Side=Left
  front brake : PMIOPort  Port=4  Side=Left
  rear brake : PMIOPort  Port=5  Side=Left
  front axle driver : PMIOPort  Port=6  Side=Left
  Longitudnal force : Outport
  Axle Torque : Outport  Port=2
  Front Axle Load : Outport  Port=3
  Reare Axle Load : Outport  Port=4
  front tire slip : Outport  Port=5
  Rear tire slip : Outport  Port=6
  wires:
  PS-Simulink Converter1/1 -> Scope/1
  PS-Simulink Converter2/1 -> Longitudnal force/1
  PS-Simulink Converter3/1 -> Axle Torque/1
  PS-Simulink Converter4/1 -> Front Axle Load/1
  PS-Simulink Converter5/1 -> Reare Axle Load/1
  PS-Simulink Converter6/1 -> front tire slip/1
  PS-Simulink Converter7/1 -> Rear tire slip/1
  connections:
  Vehicle Body/LConn2 -- PS-Simulink Converter1/LConn1
  Ideal Torque Sensor/RConn1 -- rear Tire (Magic Formula)1/LConn2
  rear Tire (Magic Formula)/LConn1 -- Vehicle Body/RConn1 -- PS-Simulink Converter5/LConn1
  PS-Simulink Converter7/LConn1 -- rear Tire (Magic Formula)/RConn1
  rear Tire (Magic Formula)1/LConn1 -- Vehicle Body/RConn2 -- PS-Simulink Converter4/LConn1
  wind/RConn1 -- Vehicle Body/LConn3
  rear Tire (Magic Formula)/RConn2 -- Hub/RConn1 -- Ideal Force Sensor/LConn1 -- Vehicle Body/LConn1
  rear Tire (Magic Formula)1/RConn1 -- PS-Simulink Converter6/LConn1
  rear brake/RConn1 -- rear Tire (Magic Formula)/LConn2
  grade/RConn1 -- Vehicle Body/RConn3
  Ideal Force Sensor/RConn1 -- rear Tire (Magic Formula)1/RConn2
  PS-Simulink Converter2/LConn1 -- Ideal Force Sensor/RConn2
  PS-Simulink Converter3/LConn1 -- Ideal Torque Sensor/RConn2
  front axle driver/RConn1 -- front brake/RConn1 -- Ideal Torque Sensor/LConn1

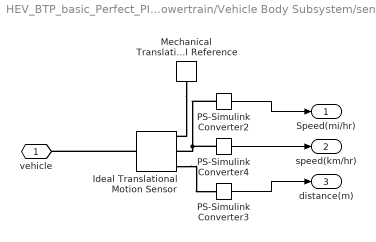
== system HEV_BTP_basic_Perfect_PID_17_1_2020/complete powertrain/Vehicle Body Subsystem/sensors ==
  Ideal Translational Motion Sensor : fl_lib/Mechanical/Mechanical Sensors/Ideal Translational Motion Sensor  offset=0 m
  Mechanical Translational Reference : fl_lib/Mechanical/Translational Elements/Mechanical Translational Reference
  PS-Simulink Converter2 : nesl_utility/PS-Simulink Converter  PhysicalDomain=network_engine_domain  SubClassName=ps_output  LeftPortType=input  RightPortType=output  PseudoPeriodic=off  Frequencies=[]  Unit=mi/hr  AffineConversion=off
  PS-Simulink Converter3 : nesl_utility/PS-Simulink Converter  PhysicalDomain=network_engine_domain  SubClassName=ps_output  LeftPortType=input  RightPortType=output  PseudoPeriodic=off  Frequencies=[]  Unit=m  AffineConversion=off
  PS-Simulink Converter4 : nesl_utility/PS-Simulink Converter  PhysicalDomain=network_engine_domain  SubClassName=ps_output  LeftPortType=input  RightPortType=output  PseudoPeriodic=off  Frequencies=[]  Unit=km/hr  AffineConversion=off
  vehicle : PMIOPort  Side=Left
  Speed(mi/hr) : Outport
  speed(km/hr) : Outport  Port=2
  "distance(m) " : Outport  Port=3
  wires:
  PS-Simulink Converter4/1 -> speed(km/hr)/1
  PS-Simulink Converter3/1 -> "distance(m) "/1
  PS-Simulink Converter2/1 -> Speed(mi/hr)/1
  connections:
  PS-Simulink Converter2/LConn1 -- PS-Simulink Converter4/LConn1 -- Ideal Translational Motion Sensor/RConn2
  Ideal Translational Motion Sensor/RConn3 -- PS-Simulink Converter3/LConn1
  Mechanical Translational Reference/LConn1 -- Ideal Translational Motion Sensor/RConn1
  Ideal Translational Motion Sensor/LConn1 -- vehicle/RConn1

== stateflow chart HEV_BTP_basic_Perfect_PID_17_1_2020/complete powertrain/Chart ==
  state GearShift
    state First
      Gear_number=1;
    state Second
      Gear_number=2;
    state Third
      Gear_number=5;
    state Fourth
      Gear_number=3;
    state Fifth
      Gear_number=4;
    (default) -> First
    First -> Second : [Vcl_Speed>13]
    Second -> First [order 1] : [Vcl_Speed<=13]
    Second -> Fourth [order 2] : [Vcl_Speed>20]
    Fourth -> Second [order 2] : [Vcl_Speed<=20]
    Third -> Fifth : [Vcl_Speed<=40]
    Fifth -> Third [order 2] : [Vcl_Speed>40]
    Fifth -> Fourth [order 1] : [Vcl_Speed<=30]
    Fourth -> Fifth [order 1] : [Vcl_Speed>30]
  (default) -> GearShift
  data: Vcl_Speed input; Gear_number output
